simulink subsystem "ApplicationMotorSwapHighPrio"  (R2024b)
settings: Solver=VariableStepAuto  StartTime=0.0  StopTime=10.0  RelTol=1e-3
values from neighbouring files (symbols this model uses):
  Ts = T_pwm    [mcbMotorSwapData.m]
undefined symbols (not defined in the file or in its folder): inverter, NumBits1, NumBits2, Per, pmsm, PosRange1, PosRange2, Slope1, Slope2, Unit
libraries: simulink x17, mcbcontrolslib x4, mcbpmsmparamestlib x3, mcbfoclib x2, mcbpmsmiflib x2, mcbpositiondecoderlib x2, mcbcomputeparameterlib x1, mcbcontrollergainlib x1
(part 1 of 2)
settings Model: Creator=The MathWorks, Inc.  LastModifiedBy=snarayan
settings RTWCC: GPUComputeCapability=3.5

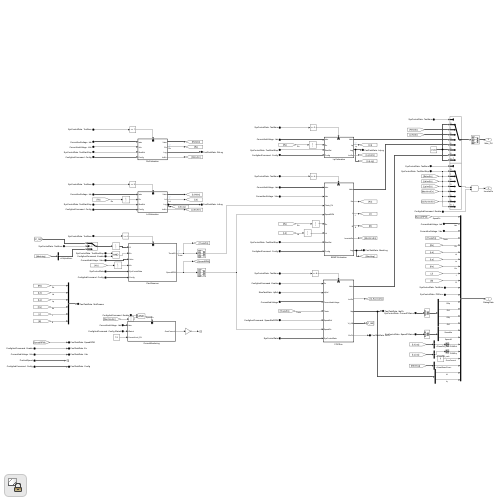
[thumbnail: Simulink's stored preview of the top-level diagram]
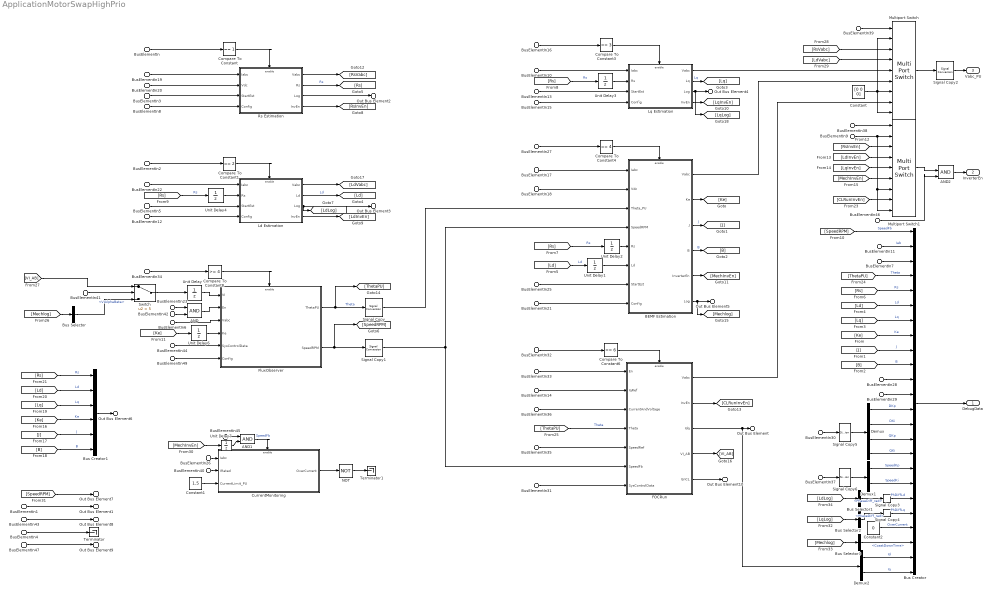
== system ApplicationMotorSwapHighPrio ==
  BusElementIn{1,33,42,45..46} (5 alike) : Inport  PortName=ConfigAndCommand  Element=Enable
  BusElementIn{8,12,15,21,47,49} (6 alike) : Inport  PortName=ConfigAndCommand  Element=Config
  BusElementIn40 : Inport  PortName=ConfigAndCommand  Element=Config.IRated
  BusElementIn35 : Inport  PortName=ConfigAndCommand  Element=SpeedRefRPM
  BusElementIn36 : Inport  Port=2  PortName=CurrentAndVoltage
  BusElementIn{10..11,17,19,22,26} (6 alike) : Inport  Port=2  PortName=CurrentAndVoltage  Element=Iab
  BusElementIn{7,18,20,43} (4 alike) : Inport  Port=2  PortName=CurrentAndVoltage  Element=Vdc
  BusElementIn6 : Inport  Port=2  PortName=CurrentAndVoltage  Element=Vabc
  BusElementIn4 : Inport  Port=3  PortName=PosAndSpeed
  BusElementIn14 : Inport  Port=4  PortName=SlowTaskData  Element=IqRef
  BusElementIn31 : Inport  Port=5  PortName=SysControlData
  BusElementIn44 : Inport  Port=5  PortName=SysControlData
  BusElementIn{,2,16,27..28,32,34,38..39,41} (10 alike) : Inport  Port=5  PortName=SysControlData  Element=TestNum
  BusElementIn29 : Inport  Port=5  PortName=SysControlData  Element=PEError
  BusElementIn{3,5,9,13,23,25} (6 alike) : Inport  Port=5  PortName=SysControlData  Element=TestStartStop
  BusElementIn30 : Inport  Port=5  PortName=SysControlData  Element=CurrentPIGains
  BusElementIn37 : Inport  Port=5  PortName=SysControlData  Element=SpeedPIGains
  AND : Logic  AllPortsSameDT=off  OutDataTypeStr=boolean
  AND1 : Logic  AllPortsSameDT=off  OutDataTypeStr=boolean
  AND2 : Logic  IconShape=distinctive  AllPortsSameDT=off  OutDataTypeStr=boolean
  BEMF Estimation : Subsystem
  Bus Creator : BusCreator  Inputs=24
  Bus Creator1 : BusCreator  Inputs=6
  Bus Selector : BusSelector  OutputSignals=VIAlphaBeta
  Bus Selector1 : BusSelector  OutputSignals=PhaseDiff_rad
  Bus Selector2 : BusSelector  OutputSignals=PhaseDiff_rad
  Bus Selector3 : BusSelector  OutputSignals=CoastDownTime
  Compare To Constant : simulink/Logic and Bit Operations/Compare To Constant  relop===  const=1  OutDataTypeStr=boolean
  Compare To Constant1 : simulink/Logic and Bit Operations/Compare To Constant  relop===  const=2  OutDataTypeStr=boolean
  Compare To Constant3 : simulink/Logic and Bit Operations/Compare To Constant  relop===  const=3  OutDataTypeStr=boolean
  Compare To Constant4 : simulink/Logic and Bit Operations/Compare To Constant  relop===  const=4  OutDataTypeStr=boolean
  Compare To Constant6 : simulink/Logic and Bit Operations/Compare To Constant  relop===  const=6  OutDataTypeStr=boolean
  Compare To Constant8 : simulink/Logic and Bit Operations/Compare To Constant  relop=>=  const=4  OutDataTypeStr=boolean
  Constant : Constant  Value=[0 0 0]  OutDataTypeStr=dataType
  Constant1 : Constant  Value=1.5  OutDataTypeStr=dataType
  Constant2 : Constant  Value=0  OutDataTypeStr=single
  CurrentMonitoring : Subsystem
  Demux : Demux
  Demux1 : Demux  Outputs=2
  Demux2 : Demux  Outputs=2
  FOCRun : Subsystem  TreatAsAtomicUnit=on
  FluxObserver : Subsystem
  Ld Estimation : Subsystem
  Lq Estimation : Subsystem
  Multiport Switch : MultiPortSwitch  DataPortOrder=Zero-based contiguous  Inputs=8  DiagnosticForDefault=None  zeroidx=on  SaturateOnIntegerOverflow=off  InputSameDT=off
  Multiport Switch1 : MultiPortSwitch  DataPortOrder=Zero-based contiguous  Inputs=8  DiagnosticForDefault=None  zeroidx=on  SaturateOnIntegerOverflow=off  InputSameDT=off
  NOT : Logic  Operator=NOT  IconShape=distinctive  AllPortsSameDT=off  OutDataTypeStr=boolean
  Rs Estimation : Subsystem
  Signal Copy{,1..6} (7 alike) : SignalConversion  OverrideOpt=on
  Switch : Switch  Criteria=u2 > Threshold  Threshold=5  SaturateOnIntegerOverflow=off  InputSameDT=off
  Terminator : Terminator
  Terminator1 : Terminator
  Unit Delay{,1..4,6..7} (7 alike) : UnitDelay  SampleTime=-1  HasFrameUpgradeWarning=on
  DebugData : Outport
  InverterEn : Outport  Port=2
  Vabc_PU : Outport  Port=3
  Out Bus Element : Outport  Port=4  PortName=FastTaskData  Element=IdqFb
  Out Bus Element1 : Outport  Port=4  PortName=FastTaskData  Element=En
  Out Bus Element2 : Outport  Port=4  PortName=FastTaskData  Element=RsLog
  Out Bus Element3 : Outport  Port=4  PortName=FastTaskData  Element=LdLog
  Out Bus Element4 : Outport  Port=4  PortName=FastTaskData  Element=LqLog
  Out Bus Element5 : Outport  Port=4  PortName=FastTaskData  Element=MechLog
  Out Bus Element6 : Outport  Port=4  PortName=FastTaskData  Element=MotParams
  Out Bus Element7 : Outport  Port=4  PortName=FastTaskData  Element=SpeedRPM
  Out Bus Element8 : Outport  Port=4  PortName=FastTaskData  Element=Vdc
  Out Bus Element9 : Outport  Port=4  PortName=FastTaskData  Element=Config
  Out Bus Element10 : Outport  Port=4  PortName=FastTaskData  Element=EnCL
  wires:
  Bus Creator/1 -> DebugData/1
  BusElementIn19/1 -> Rs Estimation/1(Iabc)
  BusElementIn20/1 -> Rs Estimation/2(Vdc)
  [Rs] -> Bus Creator/5  "Rs"
  FOCRun/3(Idq) -> Out Bus Element/1, Demux2/1
  BusElementIn11/1 -> Bus Creator/2  "Iab"
  BusElementIn14/1 -> FOCRun/2(IqRef)
  Rs Estimation/3(Log) -> Out Bus Element2/1
  BusElementIn1/1 -> Out Bus Element1/1
  BusElementIn/1 -> Compare To Constant/1
  BusElementIn22/1 -> Ld Estimation/1(Iabc)
  BusElementIn5/1 -> Ld Estimation/3(StartEst)
  BusElementIn12/1 -> Ld Estimation/4(Config)
  Ld Estimation/3(Log) -> [LdLog], Out Bus Element3/1
  Compare To Constant1/1 -> Ld Estimation/Enable
  BusElementIn2/1 -> Compare To Constant1/1
  BusElementIn3/1 -> Rs Estimation/3(StartEst)
  BusElementIn10/1 -> Lq Estimation/1(Iabc)
  BusElementIn13/1 -> Lq Estimation/3(StartEst)
  BusElementIn15/1 -> Lq Estimation/4(Config)
  Lq Estimation/3(Log) -> Out Bus Element4/1, [LqLog]
  Compare To Constant3/1 -> Lq Estimation/Enable
  BusElementIn16/1 -> Compare To Constant3/1
  [Ld] -> Bus Creator/6  "Ld"
  [Lq] -> Bus Creator/7  "Lq"
  FluxObserver/1(ThetaPU) -> Signal Copy/1, [ThetaPU]  "Theta"
  BusElementIn17/1 -> BEMF Estimation/1(Iabc)
  BusElementIn18/1 -> BEMF Estimation/2(Vdc)
  Unit Delay1/1 -> BEMF Estimation/6(Ld)
  BusElementIn25/1 -> BEMF Estimation/7(StartEst)
  BusElementIn21/1 -> BEMF Estimation/8(Config)
  [Ke] -> Bus Creator/8  "Ke"
  [J] -> Bus Creator/9  "J"
  [B] -> Bus Creator/10  "B"
  BEMF Estimation/6(Log) -> Out Bus Element5/1, [Mechlog]
  Compare To Constant4/1 -> BEMF Estimation/Enable
  BusElementIn27/1 -> Compare To Constant4/1
  BEMF Estimation/2(Ke) -> [Ke]
  BEMF Estimation/3(J) -> [J]  "J"
  BEMF Estimation/4(B) -> [B]  "B"
  Lq Estimation/2(Lq) -> [Lq]  "Lq"
  Ld Estimation/2(Ld) -> [Ld]  "Ld"
  [Ld] -> Unit Delay1/1  "Ld"
  Rs Estimation/2(Rs) -> [Rs]  "Rs"
  Unit Delay2/1 -> BEMF Estimation/5(Rs)
  [Rs] -> Unit Delay2/1  "Rs"
  Unit Delay3/1 -> Lq Estimation/2(Rs)
  [Rs] -> Unit Delay3/1  "Rs"
  Unit Delay4/1 -> Ld Estimation/2(Rs)
  [Rs] -> Unit Delay4/1  "Rs"
  FluxObserver/2(SpeedRPM) -> Signal Copy1/1, [SpeedRPM]
  BusElementIn9/1 -> Multiport Switch1/2, Multiport Switch1/7, Multiport Switch1/9
  Rs Estimation/4(InvEn) -> [RsInvEn]
  Ld Estimation/4(InvEn) -> [LdInvEn]
  Lq Estimation/4(InvEn) -> [LqInvEn]
  BEMF Estimation/5(InverterEn) -> [MechInvEn]
  BusElementIn28/1 -> Bus Creator/11
  BusElementIn29/1 -> Bus Creator/12
  [Ld] -> Bus Creator1/2  "Ld"
  [Lq] -> Bus Creator1/3  "Lq"
  [Rs] -> Bus Creator1/1  "Rs"
  [Ke] -> Bus Creator1/4  "Ke"
  [J] -> Bus Creator1/5  "J"
  [B] -> Bus Creator1/6  "B"
  Bus Creator1/1 -> Out Bus Element6/1
  Compare To Constant6/1 -> FOCRun/Enable
  BusElementIn32/1 -> Compare To Constant6/1
  FOCRun/2(InvEn) -> [CLRunInvEn]
  BusElementIn33/1 -> FOCRun/1(En)
  [ThetaPU] -> FOCRun/4(Theta)  "Theta"
  BusElementIn4/1 -> Terminator/1
  Unit Delay/1 -> FluxObserver/1(VI)
  BusElementIn23/1 -> AND/1
  [Mechlog] -> Bus Selector/1
  BusElementIn34/1 -> Compare To Constant8/1
  Compare To Constant8/1 -> FluxObserver/Enable
  Signal Copy/1 -> BEMF Estimation/3(Theta_PU)
  Signal Copy1/1 -> FOCRun/6(SpeedFb), BEMF Estimation/4(SpeedRPM)
  AND/1 -> FluxObserver/2(En)
  Switch/1 -> Unit Delay/1
  FOCRun/4(VI_AB) -> [VI_AB]
  [VI_AB] -> Switch/1
  Bus Selector/1 -> Switch/3  "<VIAlphaBeta>"
  BusElementIn41/1 -> Switch/2
  BusElementIn42/1 -> AND/2
  BusElementIn43/1 -> Out Bus Element8/1
  BusElementIn31/1 -> FOCRun/7(SysControlData)
  BusElementIn36/1 -> FOCRun/3(CurrentAndVoltage)
  [SpeedRPM] -> Out Bus Element7/1
  BusElementIn35/1 -> FOCRun/5(SpeedRef)
  BusElementIn7/1 -> Bus Creator/3
  Ld Estimation/1(Vabc) -> [LdVabc]
  FOCRun/1(Vabc) -> Multiport Switch/8
  BusElementIn30/1 -> Signal Copy5/1
  Demux/3 -> Bus Creator/15  "QKp"
  Demux/4 -> Bus Creator/16  "QKi"
  Demux/2 -> Bus Creator/14  "DKi"
  Demux/1 -> Bus Creator/13  "DKp"
  Demux1/1 -> Bus Creator/17  "SpeedKp"
  Demux1/2 -> Bus Creator/18  "SpeedKi"
  BusElementIn37/1 -> Signal Copy6/1
  Compare To Constant/1 -> Rs Estimation/Enable
  BusElementIn39/1 -> Multiport Switch/1
  Constant/1 -> Multiport Switch/7, Multiport Switch/9, Multiport Switch/2
  Multiport Switch/1 -> Signal Copy2/1
  Rs Estimation/1(Vabc) -> [RsVabc]
  [LdVabc] -> Multiport Switch/4
  [RsVabc] -> Multiport Switch/3
  Lq Estimation/1(Vabc) -> Multiport Switch/5
  BEMF Estimation/1(Vabc) -> Multiport Switch/6
  BusElementIn38/1 -> Multiport Switch1/1
  [RsInvEn] -> Multiport Switch1/3
  [LdInvEn] -> Multiport Switch1/4
  [LqInvEn] -> Multiport Switch1/5
  [MechInvEn] -> Multiport Switch1/6
  [CLRunInvEn] -> Multiport Switch1/8
  BusElementIn6/1 -> FluxObserver/3(Vabc)
  Unit Delay6/1 -> FluxObserver/4(Ke)
  [Ke] -> Unit Delay6/1
  BusElementIn44/1 -> FluxObserver/5(SysControlData)
  BusElementIn8/1 -> Rs Estimation/4(Config)
  BusElementIn26/1 -> CurrentMonitoring/1(Iabc)
  BusElementIn40/1 -> CurrentMonitoring/2(IRated)
  Constant1/1 -> CurrentMonitoring/3(CurrentLimit_PU)
  CurrentMonitoring/1(OverCurrent) -> NOT/1
  Unit Delay7/1 -> AND1/2
  BusElementIn45/1 -> AND1/1
  [MechInvEn] -> Unit Delay7/1
  AND2/1 -> InverterEn/1
  Multiport Switch1/1 -> AND2/1
  BusElementIn46/1 -> AND2/2
  BusElementIn47/1 -> Out Bus Element9/1
  Signal Copy2/1 -> Vabc_PU/1
  BusElementIn49/1 -> FluxObserver/6(Config)
  [LdLog] -> Bus Selector1/1
  Bus Selector1/1 -> Signal Copy3/1  "<PhaseDiff_rad>"
  [LqLog] -> Bus Selector2/1
  Signal Copy3/1 -> Bus Creator/19  "PhDiffLd"
  Bus Selector2/1 -> Signal Copy4/1  "<PhaseDiff_rad>"
  Signal Copy4/1 -> Bus Creator/20  "PhDiffLq"
  AND1/1 -> CurrentMonitoring/Enable  "SpeedFb"
  [SpeedRPM] -> Bus Creator/1  "SpeedFb"
  NOT/1 -> Terminator1/1
  Constant2/1 -> Bus Creator/21  "OverCurrent"
  [Mechlog] -> Bus Selector3/1
  Bus Selector3/1 -> Bus Creator/22  "<CoastDownTime>"
  Demux2/2 -> Bus Creator/24  "Iq"
  Demux2/1 -> Bus Creator/23  "Id"
  FOCRun/5(EnCL) -> Out Bus Element10/1
  [ThetaPU] -> Bus Creator/4  "Theta"
  Signal Copy5/1 -> Demux/1
  Signal Copy6/1 -> Demux1/1

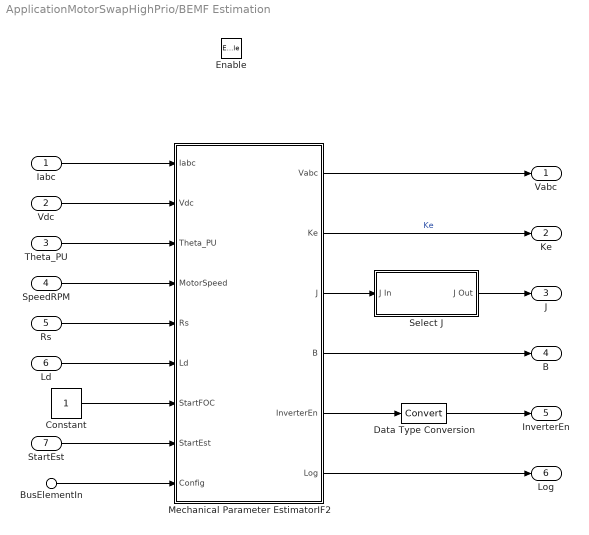
== system ApplicationMotorSwapHighPrio/BEMF Estimation ==
  Iabc : Inport
  Vdc : Inport  Port=2
  Theta_PU : Inport  Port=3
  SpeedRPM : Inport  Port=4
  Rs : Inport  Port=5
  Ld : Inport  Port=6
  StartEst : Inport  Port=7
  BusElementIn : Inport  Port=8  PortName=Config
  Enable : EnablePort  StatesWhenEnabling=reset
  Constant : Constant  OutDataTypeStr=Inherit: Inherit via back propagation
  Data Type Conversion : DataTypeConversion  SaturateOnIntegerOverflow=off  RndMeth=Floor
  Mechanical Parameter EstimatorIF2 : Subsystem  AncestorBlock=mcblib/Parameter Estimation/PMSM Parameter Estimation/Mechanical Parameter Estimator  InitFcn=|  mask(PMSM Mechanical Parameter Estimator){}
      | mcb.internal.manageMCBResource('register',gcbh);
      | mcb.internal.logDDUXData;
      mask help: mcb:ParamEstLib:PmsmKeJBEstBlkDlgDes
      mask init:
      | % mcb.internal.PMSMParameterEstimationCb();
      settings: LibrarySourceBlock=mcblib/Parameter Estimation/PMSM Parameter Estimation/Mechanical Parameter Estimator
      mask Help: eval('mcb_helpview(''pmsmmechanicalparameterestimator'')')
      mask DialogControl DescGroupVar Prompt: mcb:ParamEstLib:PmsmKeJBEstBlkDlgTitle
      mask Display:
      | fprintf('PMSM\nMechanical\nParameter\nEstimator');
      | port_label('input',1,'Iabc');
      | port_label('input',2,'Vdc');
      | port_label('input',3,'Theta');
      | port_label('input',4,'Speed');
      | port_label('input',5,'Rs');
      | port_label('input',6,'Ld');
      | port_label('input',7,'StartFOC');
      | port_label('input',8,'StartStop');
      | port_label('input',9,'Config');
      | 
      | port_label('output',1,'Vabc');
      | port_label('output',2,'Ke');
      | port_label('output',3,'J');
      | port_label('output',4,'B');
      | port_label('output',5,'InverterEn');
      | port_label('output',6,'Log');
  Select J : Subsystem  Variant=on  VariantControlMode=sim codegen switching
  Vabc : Outport
  Ke : Outport  Port=2  InitialOutput=pmsm.Ke
  J : Outport  Port=3  InitialOutput=pmsm.J
  B : Outport  Port=4  InitialOutput=pmsm.B
  InverterEn : Outport  Port=5  InitialOutput=true
  Log : Outport  Port=6
  wires:
  Constant/1 -> Mechanical Parameter EstimatorIF2/7(StartFOC)
  Mechanical Parameter EstimatorIF2/3(J) -> Select J/1(J In)
  Mechanical Parameter EstimatorIF2/4(B) -> B/1
  Select J/1(J Out) -> J/1
  Data Type Conversion/1 -> InverterEn/1
  Mechanical Parameter EstimatorIF2/6(Log) -> Log/1
  Mechanical Parameter EstimatorIF2/2(Ke) -> Ke/1  "Ke"
  Mechanical Parameter EstimatorIF2/5(InverterEn) -> Data Type Conversion/1
  Mechanical Parameter EstimatorIF2/1(Vabc) -> Vabc/1
  BusElementIn/1 -> Mechanical Parameter EstimatorIF2/9(Config)
  StartEst/1 -> Mechanical Parameter EstimatorIF2/8(StartEst)
  Ld/1 -> Mechanical Parameter EstimatorIF2/6(Ld)
  Rs/1 -> Mechanical Parameter EstimatorIF2/5(Rs)
  SpeedRPM/1 -> Mechanical Parameter EstimatorIF2/4(MotorSpeed)
  Theta_PU/1 -> Mechanical Parameter EstimatorIF2/3(Theta_PU)
  Vdc/1 -> Mechanical Parameter EstimatorIF2/2(Vdc)
  Iabc/1 -> Mechanical Parameter EstimatorIF2/1(Iabc)

== system ApplicationMotorSwapHighPrio/CurrentMonitoring ==
  Iabc : Inport
  IRated : Inport  Port=2
  CurrentLimit_PU : Inport  Port=3
  Enable : EnablePort  StatesWhenEnabling=reset
  Current and Voltage Monitoring : Subsystem
  NOT : Logic  Operator=NOT  IconShape=distinctive  AllPortsSameDT=off  OutDataTypeStr=boolean
  Unit Delay : UnitDelay  SampleTime=-1  HasFrameUpgradeWarning=on
  OverCurrent : Outport  InitialOutput=0
  wires:
  IRated/1 -> Current and Voltage Monitoring/2(IRated)
  Iabc/1 -> Current and Voltage Monitoring/1(Iabc)
  Current and Voltage Monitoring/1(OverCurrent) -> NOT/1, OverCurrent/1  "in_oc"
  CurrentLimit_PU/1 -> Current and Voltage Monitoring/3(CurrentLimit)
  NOT/1 -> Unit Delay/1
  Unit Delay/1 -> Current and Voltage Monitoring/Enable

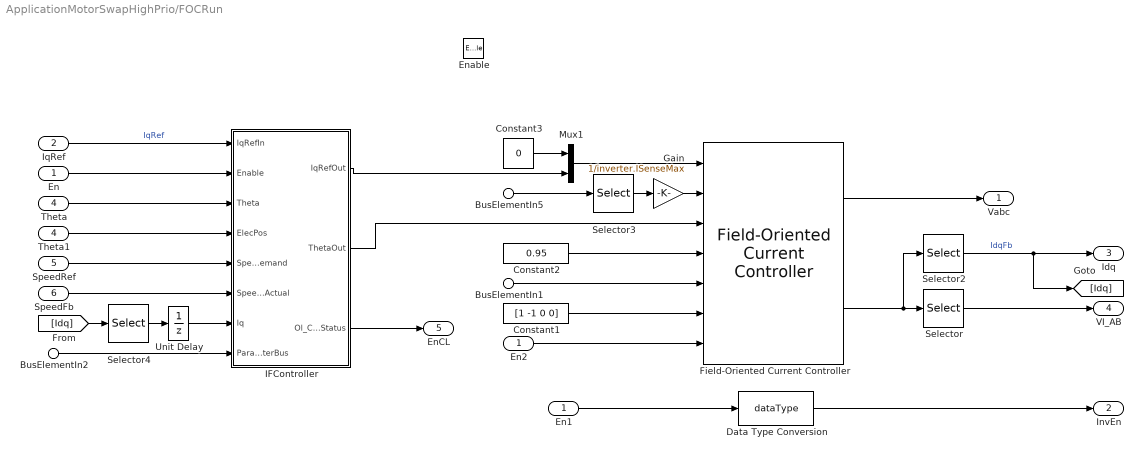
== system ApplicationMotorSwapHighPrio/FOCRun ==
  En : Inport
  IqRef : Inport  Port=2
  BusElementIn5 : Inport  Port=3  PortName=CurrentAndVoltage  Element=Iab
  Theta : Inport  Port=4
  SpeedRef : Inport  Port=5
  SpeedFb : Inport  Port=6
  BusElementIn1 : Inport  Port=7  PortName=SysControlData  Element=CurrentPIGains
  BusElementIn2 : Inport  Port=7  PortName=SysControlData  Element=IFParams
  Enable : EnablePort  StatesWhenEnabling=reset
  Constant1 : Constant  Value=[1 -1 0 0]  OutDataTypeStr=dataType
  Constant2 : Constant  Value=0.95  OutDataTypeStr=dataType
  Constant3 : Constant  Value=0  OutDataTypeStr=single
  Data Type Conversion : DataTypeConversion  OutDataTypeStr=dataType  RndMeth=Simplest  SaturateOnIntegerOverflow=off
  En1 : InportShadow
  En2 : InportShadow
  Field-Oriented Current Controller : mcbfoclib/Field-Oriented Current Controller  AngleUnit=Per-unit  NumberOfLUTPoints=1024  AxisAlignment=D-axis  SaturationMethod=D-Q equivalence  PWMMethod=SVM: space vector modulation
  Gain : Gain  Gain=1/inverter.ISenseMax  RndMeth=Simplest  OutDataTypeStr=Inherit: Same as input
  IFController : Subsystem
  Mux1 : Mux  Inputs=2
  Selector : Selector  InputPortWidth=8  IndexOptions=Index vector (dialog)  Indices=[5 6 7 8]  OutputSizes=1
  Selector2 : Selector  InputPortWidth=8  IndexOptions=Index vector (dialog)  Indices=[1 2]  OutputSizes=1
  Selector3 : Selector  InputPortWidth=3  IndexOptions=Index vector (dialog)  Indices=[1 2]  OutputSizes=1
  Selector4 : Selector  InputPortWidth=2  IndexOptions=Index vector (dialog)  Indices=[2]  OutputSizes=1
  Theta1 : InportShadow  Port=4
  Unit Delay : UnitDelay  SampleTime=-1  HasFrameUpgradeWarning=on
  Vabc : Outport
  InvEn : Outport  Port=2
  Idq : Outport  Port=3
  VI_AB : Outport  Port=4
  EnCL : Outport  Port=5
  wires:
  IFController/3(Ol_CL_Status) -> EnCL/1
  IFController/2(ThetaOut) -> Field-Oriented Current Controller/3
  IFController/1(IqRefOut) -> Mux1/2
  BusElementIn2/1 -> IFController/8(ParamterBus)
  Unit Delay/1 -> IFController/7(Iq)
  SpeedFb/1 -> IFController/6(SpeedActual)
  SpeedRef/1 -> IFController/5(SpeedDemand)
  Theta1/1 -> IFController/4(ElecPos)
  Theta/1 -> IFController/3(Theta)
  En/1 -> IFController/2(Enable)
  IqRef/1 -> IFController/1(IqRefIn)  "IqRef"
  BusElementIn1/1 -> Field-Oriented Current Controller/5
  Constant3/1 -> Mux1/1
  Mux1/1 -> Field-Oriented Current Controller/1
  Field-Oriented Current Controller/1 -> Vabc/1
  En2/1 -> Field-Oriented Current Controller/7
  Constant1/1 -> Field-Oriented Current Controller/6
  Selector4/1 -> Unit Delay/1
  [Idq] -> Selector4/1
  Selector/1 -> VI_AB/1
  BusElementIn5/1 -> Selector3/1
  Constant2/1 -> Field-Oriented Current Controller/4
  Selector2/1 -> [Idq], Idq/1  "IdqFb"
  Field-Oriented Current Controller/2 -> Selector/1, Selector2/1
  Gain/1 -> Field-Oriented Current Controller/2
  Data Type Conversion/1 -> InvEn/1
  Selector3/1 -> Gain/1
  En1/1 -> Data Type Conversion/1

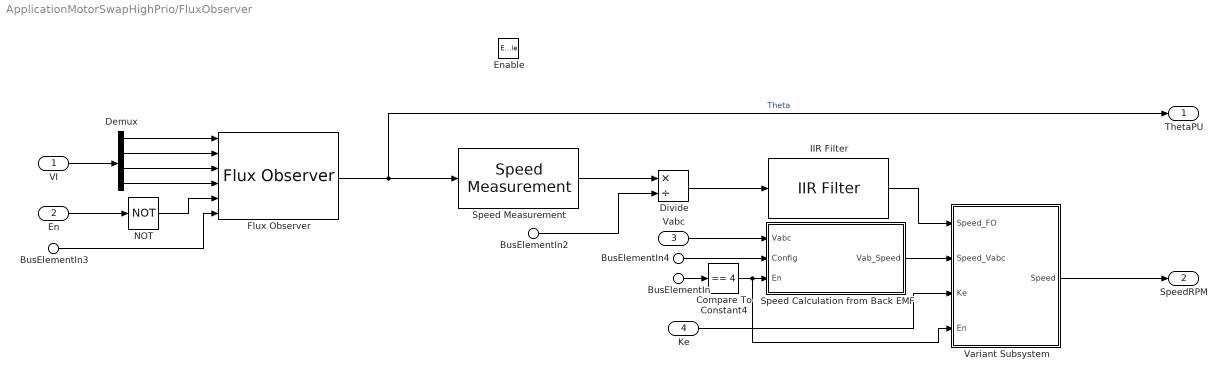
== system ApplicationMotorSwapHighPrio/FluxObserver ==
  VI : Inport
  En : Inport  Port=2
  Vabc : Inport  Port=3
  Ke : Inport  Port=4
  BusElementIn : Inport  Port=5  PortName=SysControlData  Element=TestNum
  BusElementIn3 : Inport  Port=5  PortName=SysControlData  Element=FOParams
  BusElementIn4 : Inport  Port=6  PortName=Config
  BusElementIn2 : Inport  Port=6  PortName=Config  Element=P
  Enable : EnablePort
  Compare To Constant4 : simulink/Logic and Bit Operations/Compare To Constant  relop===  const=4  OutDataTypeStr=boolean
  Demux : Demux
  Divide : Product  Inputs=*/
  Flux Observer : mcbpositiondecoderlib/Flux Observer  MotorSelection=PMSM  DataTypeSelect=off  BlockInputUnit=Per-unit  PerUnitVoltage=inverter.V_dc/sqrt(3)  PerUnitCurrent=inverter.ISenseMax  PositionSelect=on  FluxSelect=off  TorqueSelect=off  PolePairs=4  StatorResistance=0.36  StatorDAxisInductance=0.2e-3  StatorLeakageInductance=0.0068  RotorLeakageInductance=0.0068  MagnetizingInductance=0.0300  CutoffFreq=3.1863  BlockSampleTime=Ts  ParameterBusInput=on  PositionUnit=Per-unit  PositionDatatype=dataType  FluxUnit=Weber  PerUnitFlux=0.1  FluxDatatype=single  TorqueUnit=Nm  PerUnitTorque=100  TorqueDatatype=single  DataType=0
  IIR Filter : mcbcontrolslib/IIR Filter  VariantControl=Low Pass Filter  VariantSelect=Low-pass  FilterConstantInputType=Specify via dialog  Filter_constant=0.01  advancedSettings=on  Ts=Ts  cutOff_freq=25.722
  NOT : Logic  Operator=NOT  IconShape=distinctive  AllPortsSameDT=off  OutDataTypeStr=boolean
  Speed Calculation from Back EMF : Subsystem
  Speed Measurement : mcbpositiondecoderlib/Speed Measurement  PositionUnit=Per unit  PositionScalingDatatype=uint32  SpeedCalculationMode=Time interval for speed calculation  SampleTimeAsync=Ts  MaximumApplicationSpeed=1000  SpeedResolution=5e-6  DelayLength=10  MaximumMeasurableSpeed=47999  MeasurableSpeedResolution=2.2352e-05  SpeedUnit=RPM  PerUnitSpeed=1000  SpeedDataType=dataType
  Variant Subsystem : Subsystem  Variant=on  VariantControlMode=sim codegen switching
  ThetaPU : Outport
  SpeedRPM : Outport  Port=2
  wires:
  Ke/1 -> Variant Subsystem/3(Ke)
  Compare To Constant4/1 -> Speed Calculation from Back EMF/3(En), Variant Subsystem/4(En)
  BusElementIn/1 -> Compare To Constant4/1
  BusElementIn4/1 -> Speed Calculation from Back EMF/2(Config)
  Vabc/1 -> Speed Calculation from Back EMF/1(Vabc)
  Speed Calculation from Back EMF/1(Vab_Speed) -> Variant Subsystem/2(Speed_Vabc)
  IIR Filter/1 -> Variant Subsystem/1(Speed_FO)
  Variant Subsystem/1(Speed) -> SpeedRPM/1
  VI/1 -> Demux/1
  BusElementIn3/1 -> Flux Observer/6
  En/1 -> NOT/1
  NOT/1 -> Flux Observer/5
  Demux/1 -> Flux Observer/1
  Demux/4 -> Flux Observer/4
  Demux/2 -> Flux Observer/2
  Demux/3 -> Flux Observer/3
  BusElementIn2/1 -> Divide/2
  Divide/1 -> IIR Filter/1
  Speed Measurement/1 -> Divide/1
  Flux Observer/1 -> Speed Measurement/1, ThetaPU/1  "Theta"

== system ApplicationMotorSwapHighPrio/Ld Estimation ==
  Iabc : Inport
  Rs : Inport  Port=2
  StartEst : Inport  Port=3
  Config : Inport  Port=4
  Enable : EnablePort  StatesWhenEnabling=reset
  Ld Estimator : mcbpmsmparamestlib/Ld Estimator
  Vabc : Outport
  Ld : Outport  Port=2  InitialOutput=pmsm.Ld
  Log : Outport  Port=3
  InvEn : Outport  Port=4
  wires:
  Ld Estimator/2 -> Ld/1  "Ld"
  Config/1 -> Ld Estimator/4
  Ld Estimator/1 -> Vabc/1
  Rs/1 -> Ld Estimator/2
  Ld Estimator/3 -> Log/1
  StartEst/1 -> Ld Estimator/3, InvEn/1
  Iabc/1 -> Ld Estimator/1

== system ApplicationMotorSwapHighPrio/Lq Estimation ==
  Iabc : Inport
  Rs : Inport  Port=2
  StartEst : Inport  Port=3
  Config : Inport  Port=4
  Enable : EnablePort  StatesWhenEnabling=reset
  Lq Estimator : mcbpmsmparamestlib/Lq Estimator
  Vabc : Outport
  Lq : Outport  Port=2  InitialOutput=pmsm.Lq
  Log : Outport  Port=3
  InvEn : Outport  Port=4
  wires:
  StartEst/1 -> Lq Estimator/3, InvEn/1
  Lq Estimator/3 -> Log/1
  Rs/1 -> Lq Estimator/2
  Lq Estimator/1 -> Vabc/1
  Config/1 -> Lq Estimator/4
  Lq Estimator/2 -> Lq/1
  Iabc/1 -> Lq Estimator/1

== system ApplicationMotorSwapHighPrio/Rs Estimation ==
  Iabc : Inport
  Vdc : Inport  Port=2
  StartEst : Inport  Port=3
  Config : Inport  Port=4
  Enable : EnablePort  StatesWhenEnabling=reset
  Rs Estimator : mcbpmsmparamestlib/Rs Estimator
  Vabc : Outport
  Rs : Outport  Port=2  InitialOutput=pmsm.Rs
  Log : Outport  Port=3
  InvEn : Outport  Port=4
  wires:
  Rs Estimator/1 -> Vabc/1
  Iabc/1 -> Rs Estimator/1
  Rs Estimator/3 -> Log/1
  Vdc/1 -> Rs Estimator/2
  Config/1 -> Rs Estimator/4
  StartEst/1 -> InvEn/1, Rs Estimator/3
  Rs Estimator/2 -> Rs/1  "Rs"

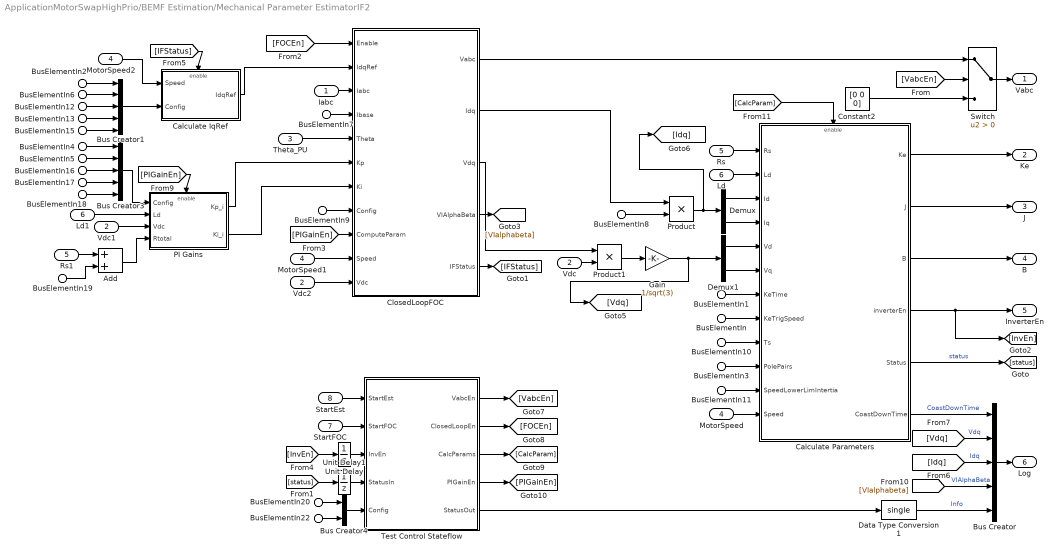
== system ApplicationMotorSwapHighPrio/BEMF Estimation/Mechanical Parameter EstimatorIF2 ==
  Iabc : Inport  OutDataTypeStr=single
  Vdc : Inport  Port=2  OutDataTypeStr=single
  Theta_PU : Inport  Port=3  OutDataTypeStr=single
  MotorSpeed : Inport  Port=4  OutDataTypeStr=single
  Rs : Inport  Port=5  OutDataTypeStr=single
  Ld : Inport  Port=6  OutDataTypeStr=single
  StartFOC : Inport  Port=7
  StartEst : Inport  Port=8
  BusElementIn9 : Inport  Port=9  PortName=Config
  BusElementIn10 : Inport  Port=9  PortName=Config  Element=Ts
  BusElementIn16 : Inport  Port=9  PortName=Config  Element=Ts
  BusElementIn20 : Inport  Port=9  PortName=Config  Element=Ts
  BusElementIn4 : Inport  Port=9  PortName=Config  Element=Kp
  BusElementIn5 : Inport  Port=9  PortName=Config  Element=Ki
  BusElementIn6 : Inport  Port=9  PortName=Config  Element=IRated
  BusElementIn1 : Inport  Port=9  PortName=Config  Element=KeTime
  BusElementIn22 : Inport  Port=9  PortName=Config  Element=KeTime
  BusElementIn3 : Inport  Port=9  PortName=Config  Element=P
  BusElementIn11 : Inport  Port=9  PortName=Config  Element=JSpeedLow
  BusElementIn2 : Inport  Port=9  PortName=Config  Element=IqRefFoc
  BusElementIn{7..8,12,18} (4 alike) : Inport  Port=9  PortName=Config  Element=ImaxInverter
  BusElementIn : Inport  Port=9  PortName=Config  Element=KeSpeed
  BusElementIn13 : Inport  Port=9  PortName=Config  Element=KeSpeed
  BusElementIn15 : Inport  Port=9  PortName=Config  Element=NRated
  BusElementIn17 : Inport  Port=9  PortName=Config  Element=KpKiInputEnable
  BusElementIn19 : Inport  Port=9  PortName=Config  Element=RBoard
  Add : Sum  RndMeth=Simplest  OutDataTypeStr=Inherit: Same as first input
  Bus Creator : BusCreator  Inputs=5
  Bus Creator1 : BusCreator  Inputs=5
  Bus Creator3 : BusCreator  Inputs=5
  Bus Creator4 : BusCreator  Inputs=2
  Calculate IqRef : Subsystem
  Calculate Parameters : Subsystem
  ClosedLoopFOC : Subsystem
  Constant2 : Constant  Value=[0 0 0]  OutDataTypeStr=single
  Data Type Conversion1 : DataTypeConversion  OutDataTypeStr=single  RndMeth=Simplest  SaturateOnIntegerOverflow=off
  Demux : Demux  Outputs=2
  Demux1 : Demux  Outputs=2
  Gain : Gain  Gain=1/sqrt(3)  RndMeth=Simplest  OutDataTypeStr=Inherit: Same as input
  Ld1 : InportShadow  Port=6  OutDataTypeStr=single
  MotorSpeed1 : InportShadow  Port=4  OutDataTypeStr=single
  MotorSpeed2 : InportShadow  Port=4  OutDataTypeStr=single
  PI Gains : Subsystem
  Product : Product  RndMeth=Simplest  OutDataTypeStr=Inherit: Same as first input
  Product1 : Product  RndMeth=Simplest  OutDataTypeStr=Inherit: Same as first input
  Rs1 : InportShadow  Port=5  OutDataTypeStr=single
  Switch : Switch  Criteria=u2 > Threshold  SaturateOnIntegerOverflow=off  InputSameDT=off
  Test Control Stateflow : Subsystem
  Unit Delay : UnitDelay  SampleTime=-1  HasFrameUpgradeWarning=on
  Unit Delay1 : UnitDelay  SampleTime=-1  HasFrameUpgradeWarning=on
  Vdc1 : InportShadow  Port=2  OutDataTypeStr=single
  Vdc2 : InportShadow  Port=2  OutDataTypeStr=single
  Vabc : Outport  InitialOutput=[0 0 0]
  Ke : Outport  Port=2
  J : Outport  Port=3
  B : Outport  Port=4
  InverterEn : Outport  Port=5
  Log : Outport  Port=6
  wires:
  Data Type Conversion1/1 -> Bus Creator/5  "Info"
  [PIGainEn] -> PI Gains/Enable
  Test Control Stateflow/4(PIGainEn) -> [PIGainEn]
  Test Control Stateflow/2(ClosedLoopEn) -> [FOCEn]
  Iabc/1 -> ClosedLoopFOC/3(Iabc)
  [Vdq] -> Bus Creator/2  "Vdq"
  [Idq] -> Bus Creator/3  "Idq"
  BusElementIn19/1 -> Add/2
  Rs1/1 -> Add/1
  Add/1 -> PI Gains/4(Rtotal)
  Vdc1/1 -> PI Gains/3(Vdc)
  Ld1/1 -> PI Gains/2(Ld)
  BusElementIn18/1 -> Bus Creator3/5
  [VabcEn] -> Switch/2
  [InvEn] -> Unit Delay/1
  BusElementIn/1 -> Calculate Parameters/8(KeTrigSpeed)
  ClosedLoopFOC/4(VIAlphaBeta) -> [VIalphabeta]
  Calculate Parameters/6(CoastDownTime) -> Bus Creator/1  "CoastDownTime"
  BusElementIn11/1 -> Calculate Parameters/11(SpeedLowerLimIntertia)
  Calculate Parameters/4(inverterEn) -> InverterEn/1, [InvEn]
  Rs/1 -> Calculate Parameters/1(Rs)
  Calculate Parameters/3(B) -> B/1
  BusElementIn10/1 -> Calculate Parameters/9(Ts)
  Bus Creator/1 -> Log/1
  Calculate Parameters/5(Status) -> [status]  "status"
  Demux/2 -> Calculate Parameters/4(Iq)
  BusElementIn1/1 -> Calculate Parameters/7(KeTime)
  Calculate Parameters/2(J) -> J/1
  Ld/1 -> Calculate Parameters/2(Ld)
  Demux1/2 -> Calculate Parameters/6(Vq)
  Demux1/1 -> Calculate Parameters/5(Vd)
  Demux/1 -> Calculate Parameters/3(Id)
  MotorSpeed/1 -> Calculate Parameters/12(Speed)
  BusElementIn3/1 -> Calculate Parameters/10(PolePairs)
  Calculate Parameters/1(Ke) -> Ke/1
  ClosedLoopFOC/2(Idq) -> Product/1
  Product/1 -> Demux/1, [Idq]
  Vdc/1 -> Product1/2
  ClosedLoopFOC/3(Vdq) -> Product1/1
  Product1/1 -> Gain/1
  Gain/1 -> Demux1/1, [Vdq]
  Theta_PU/1 -> ClosedLoopFOC/5(Theta)
  Switch/1 -> Vabc/1
  Constant2/1 -> Switch/3
  MotorSpeed2/1 -> Calculate IqRef/1(Speed)
  Calculate IqRef/1(IdqRef) -> ClosedLoopFOC/2(IdqRef)
  PI Gains/1(Kp_i) -> ClosedLoopFOC/6(Kp)
  PI Gains/2(Ki_i) -> ClosedLoopFOC/7(Ki)
  BusElementIn12/1 -> Bus Creator1/3
  BusElementIn13/1 -> Bus Creator1/4
  BusElementIn6/1 -> Bus Creator1/2
  BusElementIn2/1 -> Bus Creator1/1
  BusElementIn15/1 -> Bus Creator1/5
  Bus Creator1/1 -> Calculate IqRef/2(Config)
  BusElementIn8/1 -> Product/2
  BusElementIn4/1 -> Bus Creator3/1
  BusElementIn5/1 -> Bus Creator3/2
  BusElementIn16/1 -> Bus Creator3/3
  BusElementIn17/1 -> Bus Creator3/4
  Bus Creator3/1 -> PI Gains/1(Config)
  BusElementIn7/1 -> ClosedLoopFOC/4(Ibase)
  StartEst/1 -> Test Control Stateflow/1(StartEst)
  StartFOC/1 -> Test Control Stateflow/2(StartFOC)
  Unit Delay/1 -> Test Control Stateflow/3(InvEn)
  [status] -> Unit Delay1/1
  Unit Delay1/1 -> Test Control Stateflow/4(StatusIn)
  Bus Creator4/1 -> Test Control Stateflow/5(Config)
  BusElementIn22/1 -> Bus Creator4/2
  BusElementIn20/1 -> Bus Creator4/1
  Test Control Stateflow/5(StatusOut) -> Data Type Conversion1/1
  Test Control Stateflow/1(VabcEn) -> [VabcEn]
  [FOCEn] -> ClosedLoopFOC/1(Enable)
  Test Control Stateflow/3(CalcParams) -> [CalcParam]
  [CalcParam] -> Calculate Parameters/Enable
  BusElementIn9/1 -> ClosedLoopFOC/8(Config)
  [VIalphabeta] -> Bus Creator/4  "VIAlphaBeta"
  ClosedLoopFOC/1(Vabc) -> Switch/1
  [PIGainEn] -> ClosedLoopFOC/9(ComputeParam)
  MotorSpeed1/1 -> ClosedLoopFOC/10(Speed)
  Vdc2/1 -> ClosedLoopFOC/11(Vdc)
  ClosedLoopFOC/5(IFStatus) -> [IFStatus]
  [IFStatus] -> Calculate IqRef/Enable

== system ApplicationMotorSwapHighPrio/BEMF Estimation/Select J ==
  note: 1) Add Subsystem or Model blocks as valid variant choices.
      | 2) You cannot connect blocks at this level. At simulation, connectivity is automatically
      | determined, based on the active variant and port name matching.
  J In : Inport
  Codegen : Subsystem  VariantControl=(codegen)
  Sim : Subsystem  VariantControl=(sim)
  J Out : Outport

== system ApplicationMotorSwapHighPrio/CurrentMonitoring/Current and Voltage Monitoring ==
  note: As a ratio of motor rated current
  Iabc : Inport
  IRated : Inport  Port=2
  CurrentLimit : Inport  Port=3
  Enable : EnablePort
  Abs : Abs  SaturateOnIntegerOverflow=off
  Demux : Demux  Outputs=2
  Divide : Product  Inputs=*/  RndMeth=Simplest  OutDataTypeStr=Inherit: Same as first input
  GreaterThan : RelationalOperator  Operator=>  OutDataTypeStr=boolean  RndMeth=Simplest  InputSameDT=off
  GreaterThan1 : RelationalOperator  Operator=>  OutDataTypeStr=boolean  RndMeth=Simplest  InputSameDT=off
  IIR Filter : mcbcontrolslib/IIR Filter  VariantControl=Low Pass Filter  VariantSelect=Low-pass  FilterConstantInputType=Specify via dialog  Filter_constant=0.01  advancedSettings=off  Ts=50e-6  cutOff_freq=32.1525
  OR : Logic  Operator=OR  IconShape=distinctive  AllPortsSameDT=off  OutDataTypeStr=boolean
  Selector : Selector  InputPortWidth=3  IndexOptions=Index vector (dialog)  Indices=[1 2]  OutputSizes=1
  OverCurrent : Outport
  wires:
  Selector/1 -> Divide/1
  Iabc/1 -> Selector/1
  IRated/1 -> Divide/2
  Demux/1 -> GreaterThan/1
  IIR Filter/1 -> Abs/1
  Divide/1 -> IIR Filter/1
  Abs/1 -> Demux/1
  OR/1 -> OverCurrent/1
  Demux/2 -> GreaterThan1/1
  CurrentLimit/1 -> GreaterThan/2, GreaterThan1/2
  GreaterThan/1 -> OR/1
  GreaterThan1/1 -> OR/2

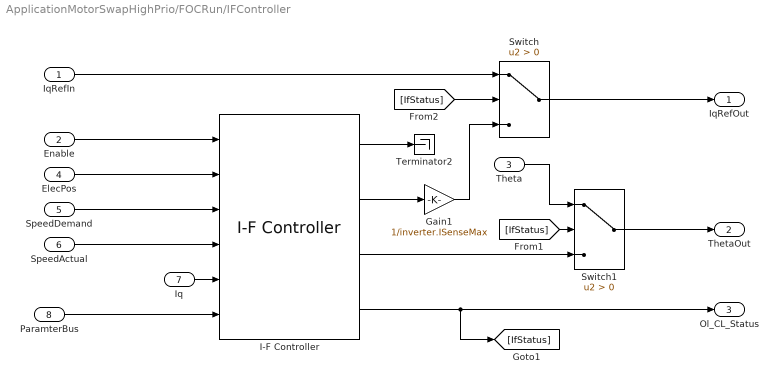
== system ApplicationMotorSwapHighPrio/FOCRun/IFController ==
  IqRefIn : Inport
  Enable : Inport  Port=2
  Theta : Inport  Port=3
  ElecPos : Inport  Port=4
  SpeedDemand : Inport  Port=5
  SpeedActual : Inport  Port=6
  Iq : Inport  Port=7
  ParamterBus : Inport  Port=8
  Gain1 : Gain  Gain=1/inverter.ISenseMax  RndMeth=Simplest  OutDataTypeStr=Inherit: Same as input
  I-F Controller : mcbpmsmiflib/I-F Controller  EnableSpeedDamp=off  PolePairs=4  PositionUnit=Per-unit  SpeedUnit=RPM  PerUnitSpeed=6000  CurrentUnit=SI unit  TempCurrentUnit=SI unit  MaxStatorCurrent=21.4286  BlkSampleTime=Ts  ParameterBusInput=on  OlClSpeed=400  ClOlSpeed=200  MaxStartingCurrent=7  MaxAcceleration=960  CurrentDownSlope=11  IdleTime=1  Angle=10 * pi / 180  VoltageUnit=SI unit  TempVoltageUnit=SI unit  MaxStatorVoltage=13.8564  DampCoeff=2.6172
  Switch : Switch  Criteria=u2 > Threshold  SaturateOnIntegerOverflow=off  InputSameDT=off
  Switch1 : Switch  Criteria=u2 > Threshold  SaturateOnIntegerOverflow=off  InputSameDT=off
  Terminator2 : Terminator
  IqRefOut : Outport
  ThetaOut : Outport  Port=2
  Ol_CL_Status : Outport  Port=3
  wires:
  IqRefIn/1 -> Switch/1
  ParamterBus/1 -> I-F Controller/6
  Switch/1 -> IqRefOut/1
  SpeedDemand/1 -> I-F Controller/3
  Switch1/1 -> ThetaOut/1
  SpeedActual/1 -> I-F Controller/4
  Iq/1 -> I-F Controller/5
  [IfStatus] -> Switch1/2
  I-F Controller/3 -> Switch1/3
  ElecPos/1 -> I-F Controller/2
  I-F Controller/4 -> [IfStatus], Ol_CL_Status/1
  I-F Controller/2 -> Gain1/1
  I-F Controller/1 -> Terminator2/1
  Theta/1 -> Switch1/1
  Enable/1 -> I-F Controller/1
  [IfStatus] -> Switch/2
  Gain1/1 -> Switch/3

== system ApplicationMotorSwapHighPrio/FluxObserver/Speed Calculation from Back EMF ==
  Vabc : Inport
  BusElementIn2 : Inport  Port=2  PortName=Config  Element=NRated
  BusElementIn3 : Inport  Port=2  PortName=Config  Element=P
  En : Inport  Port=3
  Demux : Demux  Outputs=3
  Speed Measurement : Subsystem
  Terminator : Terminator
  Vab_Speed : Outport
  wires:
  En/1 -> Speed Measurement/Enable
  Vabc/1 -> Demux/1
  Demux/2 -> Speed Measurement/2(Vb)
  Demux/1 -> Speed Measurement/1(Va)
  Speed Measurement/1(Speed) -> Vab_Speed/1
  BusElementIn3/1 -> Speed Measurement/4(p)
  Demux/3 -> Terminator/1
  BusElementIn2/1 -> Speed Measurement/3(SpeedRated)

== system ApplicationMotorSwapHighPrio/FluxObserver/Variant Subsystem ==
  Speed_FO : Inport
  Speed_Vabc : Inport  Port=2
  Ke : Inport  Port=3
  En : Inport  Port=4
  Codegen : Subsystem  VariantControl=(codegen)
  Sim : Subsystem  VariantControl=(sim)
  Speed : Outport

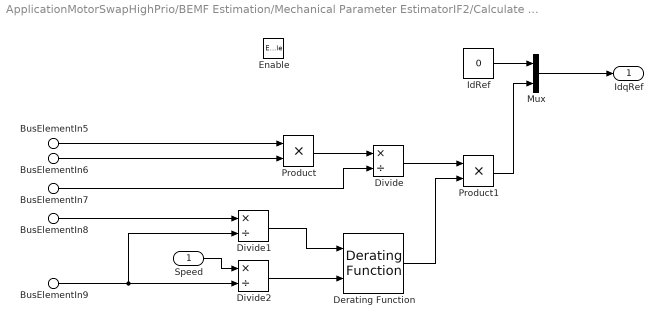
== system ApplicationMotorSwapHighPrio/BEMF Estimation/Mechanical Parameter EstimatorIF2/Calculate IqRef ==
  Speed : Inport
  BusElementIn5 : Inport  Port=2  PortName=Config  Element=IqRefFoc
  BusElementIn6 : Inport  Port=2  PortName=Config  Element=IRated
  BusElementIn7 : Inport  Port=2  PortName=Config  Element=ImaxInverter
  BusElementIn8 : Inport  Port=2  PortName=Config  Element=KeSpeed
  BusElementIn9 : Inport  Port=2  PortName=Config  Element=NRated
  Enable : EnablePort  StatesWhenEnabling=reset
  Derating Function : mcbcontrolslib/Derating Function  x=0.9
  Divide : Product  Inputs=*/  RndMeth=Simplest  OutDataTypeStr=Inherit: Same as first input
  Divide1 : Product  Inputs=*/  RndMeth=Simplest  OutDataTypeStr=Inherit: Same as first input
  Divide2 : Product  Inputs=*/  RndMeth=Simplest  OutDataTypeStr=Inherit: Same as first input
  IdRef : Constant  Value=0  OutDataTypeStr=single
  Mux : Mux  Inputs=2
  Product : Product  RndMeth=Simplest  OutDataTypeStr=Inherit: Same as first input
  Product1 : Product  RndMeth=Simplest  OutDataTypeStr=Inherit: Same as first input
  IdqRef : Outport
  wires:
  BusElementIn5/1 -> Product/1
  IdRef/1 -> Mux/1
  Mux/1 -> IdqRef/1
  BusElementIn6/1 -> Product/2
  Product/1 -> Divide/1
  BusElementIn7/1 -> Divide/2
  Divide/1 -> Product1/1
  Derating Function/1 -> Product1/2
  Speed/1 -> Divide2/1
  BusElementIn8/1 -> Divide1/1
  Divide1/1 -> Derating Function/1
  Divide2/1 -> Derating Function/2
  BusElementIn9/1 -> Divide1/2, Divide2/2
  Product1/1 -> Mux/2

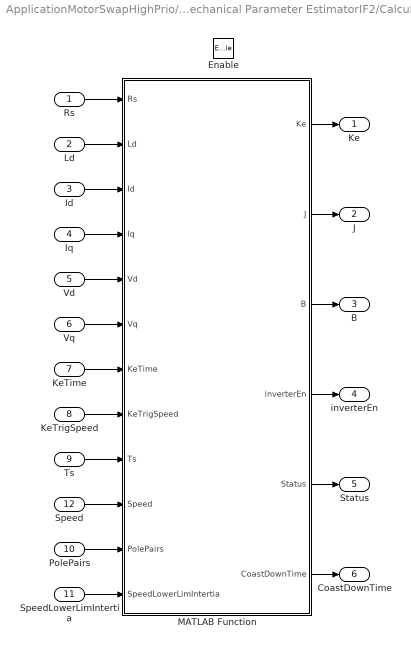
== system ApplicationMotorSwapHighPrio/BEMF Estimation/Mechanical Parameter EstimatorIF2/Calculate Parameters ==
  Rs : Inport
  Ld : Inport  Port=2
  Id : Inport  Port=3
  Iq : Inport  Port=4
  Vd : Inport  Port=5
  Vq : Inport  Port=6
  KeTime : Inport  Port=7
  KeTrigSpeed : Inport  Port=8
  Ts : Inport  Port=9
  PolePairs : Inport  Port=10
  SpeedLowerLimIntertia : Inport  Port=11
  Speed : Inport  Port=12
  Enable : EnablePort  StatesWhenEnabling=reset
  MATLAB Function : MATLAB Function  TreatAsAtomicUnit=on
  Ke : Outport
  J : Outport  Port=2
  B : Outport  Port=3
  inverterEn : Outport  Port=4  InitialOutput=1
  Status : Outport  Port=5  InitialOutput=1
  CoastDownTime : Outport  Port=6  InitialOutput=1
  wires:
  KeTrigSpeed/1 -> MATLAB Function/8(KeTrigSpeed)
  Speed/1 -> MATLAB Function/10(Speed)
  Ts/1 -> MATLAB Function/9(Ts)
  KeTime/1 -> MATLAB Function/7(KeTime)
  Vq/1 -> MATLAB Function/6(Vq)
  Vd/1 -> MATLAB Function/5(Vd)
  Iq/1 -> MATLAB Function/4(Iq)
  Id/1 -> MATLAB Function/3(Id)
  SpeedLowerLimIntertia/1 -> MATLAB Function/12(SpeedLowerLimIntertia)
  Ld/1 -> MATLAB Function/2(Ld)
  PolePairs/1 -> MATLAB Function/11(PolePairs)
  Rs/1 -> MATLAB Function/1(Rs)
  MATLAB Function/3(B) -> B/1
  MATLAB Function/1(Ke) -> Ke/1
  MATLAB Function/2(J) -> J/1
  MATLAB Function/4(inverterEn) -> inverterEn/1
  MATLAB Function/5(Status) -> Status/1
  MATLAB Function/6(CoastDownTime) -> CoastDownTime/1

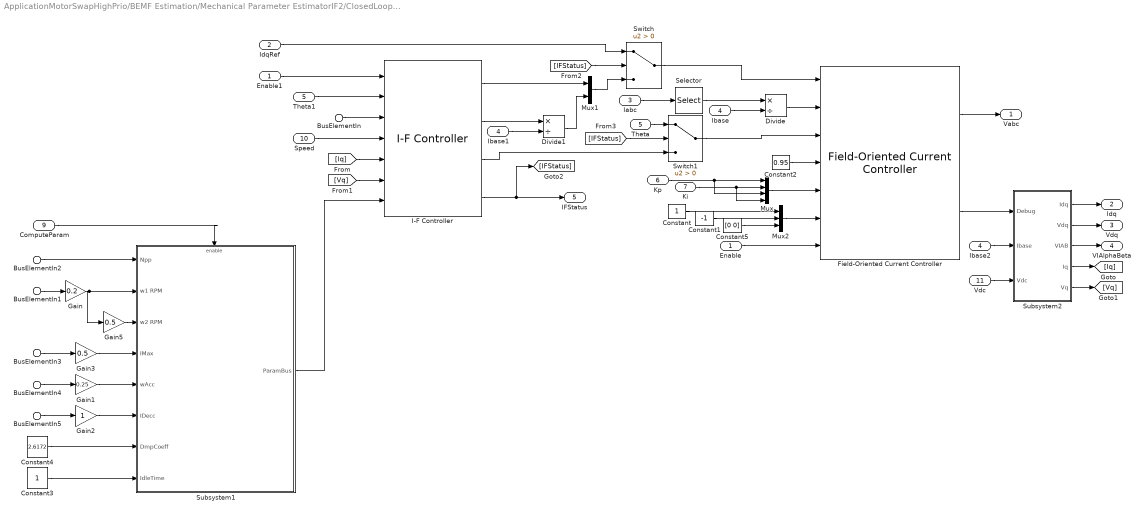
== system ApplicationMotorSwapHighPrio/BEMF Estimation/Mechanical Parameter EstimatorIF2/ClosedLoopFOC ==
  Enable : Inport
  IdqRef : Inport  Port=2
  Iabc : Inport  Port=3
  Ibase : Inport  Port=4
  Theta : Inport  Port=5
  Kp : Inport  Port=6
  Ki : Inport  Port=7
  BusElementIn : Inport  Port=8  PortName=Config  Element=KeSpeed
  BusElementIn1 : Inport  Port=8  PortName=Config  Element=NRated
  BusElementIn4 : Inport  Port=8  PortName=Config  Element=NRated
  BusElementIn2 : Inport  Port=8  PortName=Config  Element=P
  BusElementIn3 : Inport  Port=8  PortName=Config  Element=IRated
  BusElementIn5 : Inport  Port=8  PortName=Config  Element=IRated
  ComputeParam : Inport  Port=9
  Speed : Inport  Port=10
  Vdc : Inport  Port=11
  Constant : Constant  OutDataTypeStr=single
  Constant1 : Constant  Value=-1  OutDataTypeStr=single
  Constant2 : Constant  Value=0.95  OutDataTypeStr=single
  Constant3 : Constant  OutDataTypeStr=single
  Constant4 : Constant  Value=2.6172  OutDataTypeStr=single
  Constant5 : Constant  Value=[0 0]  OutDataTypeStr=single
  Divide : Product  Inputs=*/
  Divide1 : Product  Inputs=*/
  Enable1 : InportShadow
  Field-Oriented Current Controller : mcbfoclib/Field-Oriented Current Controller  AngleUnit=Per-unit  NumberOfLUTPoints=1024  AxisAlignment=D-axis  SaturationMethod=D-Q equivalence  PWMMethod=SVM: space vector modulation
  Gain : Gain  Gain=0.2  RndMeth=Simplest  OutDataTypeStr=Inherit: Same as input
  Gain1 : Gain  Gain=0.25  RndMeth=Simplest  OutDataTypeStr=Inherit: Same as input
  Gain2 : Gain  RndMeth=Simplest  OutDataTypeStr=Inherit: Same as input
  Gain3 : Gain  Gain=0.5  RndMeth=Simplest  OutDataTypeStr=Inherit: Same as input
  Gain5 : Gain  Gain=0.5  RndMeth=Simplest  OutDataTypeStr=Inherit: Same as input
  I-F Controller : mcbpmsmiflib/I-F Controller  EnableSpeedDamp=on  PolePairs=4  PositionUnit=Per-unit  SpeedUnit=RPM  PerUnitSpeed=6000  CurrentUnit=SI unit  TempCurrentUnit=SI unit  MaxStatorCurrent=21.4286  BlkSampleTime=Ts  ParameterBusInput=on  OlClSpeed=410.7  ClOlSpeed=287.49  MaxStartingCurrent=6.39  MaxAcceleration=960  CurrentDownSlope=111.8250  IdleTime=1  Angle=5 * 2 * pi / 360  VoltageUnit=SI unit  TempVoltageUnit=SI unit  MaxStatorVoltage=13.8564  DampCoeff=2.6172
  Ibase1 : InportShadow  Port=4
  Ibase2 : InportShadow  Port=4
  Mux : Mux
  Mux1 : Mux  Inputs=2
  Mux2 : Mux  Inputs=3
  Selector : Selector  InputPortWidth=3  IndexOptions=Index vector (dialog)  Indices=[1 2]  OutputSizes=1
  Subsystem1 : Subsystem
  Subsystem2 : Subsystem
  Switch : Switch  Criteria=u2 > Threshold  SaturateOnIntegerOverflow=off  InputSameDT=off
  Switch1 : Switch  Criteria=u2 > Threshold  SaturateOnIntegerOverflow=off  InputSameDT=off
  Theta1 : InportShadow  Port=5
  Vabc : Outport
  Idq : Outport  Port=2
  Vdq : Outport  Port=3
  VIAlphaBeta : Outport  Port=4
  IFStatus : Outport  Port=5
  wires:
  Mux/1 -> Field-Oriented Current Controller/5
  Ki/1 -> Mux/2, Mux/4
  Enable/1 -> Field-Oriented Current Controller/7
  Constant2/1 -> Field-Oriented Current Controller/4
  Constant1/1 -> Mux2/2
  Kp/1 -> Mux/1, Mux/3
  Field-Oriented Current Controller/1 -> Vabc/1
  Ibase/1 -> Divide/2
  Iabc/1 -> Selector/1
  Divide/1 -> Field-Oriented Current Controller/2
  Selector/1 -> Divide/1
  Constant/1 -> Mux2/1
  Constant5/1 -> Mux2/3
  Mux2/1 -> Field-Oriented Current Controller/6
  I-F Controller/1 -> Mux1/1
  Theta1/1 -> I-F Controller/2
  Enable1/1 -> I-F Controller/1
  BusElementIn/1 -> I-F Controller/3
  Mux1/1 -> Switch/3
  IdqRef/1 -> Switch/1
  Switch/1 -> Field-Oriented Current Controller/1
  I-F Controller/3 -> Switch1/3
  I-F Controller/4 -> [IFStatus], IFStatus/1
  Theta/1 -> Switch1/1
  Switch1/1 -> Field-Oriented Current Controller/3
  BusElementIn1/1 -> Gain/1
  BusElementIn4/1 -> Gain1/1
  BusElementIn5/1 -> Gain2/1
  BusElementIn2/1 -> Subsystem1/1(Npp)
  Gain/1 -> Gain5/1, Subsystem1/2(w1 RPM)
  BusElementIn3/1 -> Gain3/1
  Gain1/1 -> Subsystem1/5(wAcc)
  Gain2/1 -> Subsystem1/6(IDecc)
  Subsystem1/1(ParamBus) -> I-F Controller/7
  ComputeParam/1 -> Subsystem1/Enable
  Speed/1 -> I-F Controller/4
  Ibase1/1 -> Divide1/2
  I-F Controller/2 -> Divide1/1
  Divide1/1 -> Mux1/2
  Gain3/1 -> Subsystem1/4(IMax)
  Constant4/1 -> Subsystem1/7(DmpCoeff)
  Constant3/1 -> Subsystem1/8(IdleTime)
  Gain5/1 -> Subsystem1/3(w2 RPM)
  [Iq] -> I-F Controller/5
  [Vq] -> I-F Controller/6
  Field-Oriented Current Controller/2 -> Subsystem2/1(Debug)
  Ibase2/1 -> Subsystem2/2(Ibase)
  Vdc/1 -> Subsystem2/3(Vdc)
  Subsystem2/1(Idq) -> Idq/1
  Subsystem2/2(Vdq) -> Vdq/1
  Subsystem2/3(VIAB) -> VIAlphaBeta/1
  Subsystem2/4(Iq) -> [Iq]
  Subsystem2/5(Vq) -> [Vq]
  [IFStatus] -> Switch/2
  [IFStatus] -> Switch1/2

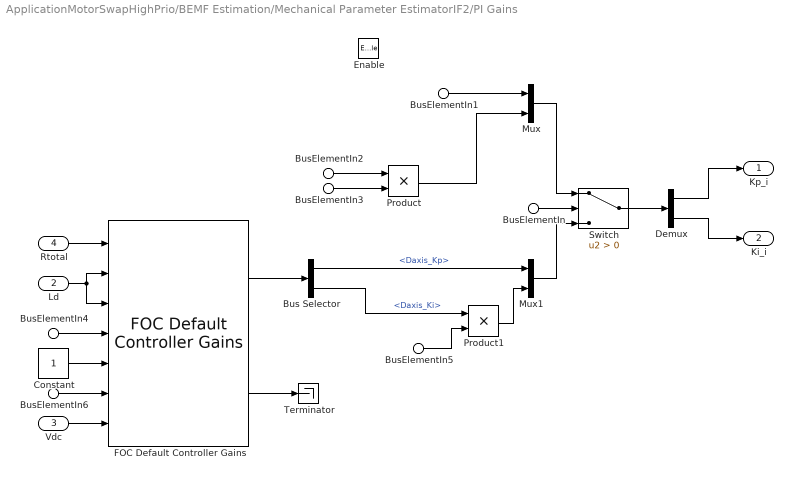
== system ApplicationMotorSwapHighPrio/BEMF Estimation/Mechanical Parameter EstimatorIF2/PI Gains ==
  BusElementIn1 : Inport  PortName=Config  Element=Kp
  BusElementIn2 : Inport  PortName=Config  Element=Ki
  BusElementIn3 : Inport  PortName=Config  Element=Ts
  BusElementIn5 : Inport  PortName=Config  Element=Ts
  BusElementIn4 : Inport  PortName=Config  Element=Ts
  BusElementIn : Inport  PortName=Config  Element=KpKiInputEnable
  BusElementIn6 : Inport  PortName=Config  Element=ImaxInverter
  Ld : Inport  Port=2  OutDataTypeStr=single
  Vdc : Inport  Port=3  OutDataTypeStr=single
  Rtotal : Inport  Port=4  OutDataTypeStr=single
  Enable : EnablePort
  Bus Selector : BusSelector  OutputSignals=Daxis_Kp,Daxis_Ki
  Constant : Constant  OutDataTypeStr=Inherit: Inherit via back propagation
  Demux : Demux  Outputs=2
  FOC Default Controller Gains : mcbcontrollergainlib/FOC Default Controller Gains  motorSelection=PMSM  unitType=Per-Unit  outCurrentControlGain=on  outFWCGain=off  outSpeedControlGain=off  externalDelay=off  currentSensorDelay=50e-6  speedSensorDelay=50e-6  speedFilterDelay=0.02
  Mux : Mux  Inputs=2
  Mux1 : Mux  Inputs=2
  Product : Product  RndMeth=Simplest  OutDataTypeStr=Inherit: Same as first input
  Product1 : Product  RndMeth=Simplest  OutDataTypeStr=Inherit: Same as first input
  Switch : Switch  Criteria=u2 > Threshold  SaturateOnIntegerOverflow=off  InputSameDT=off
  Terminator : Terminator
  Kp_i : Outport
  Ki_i : Outport  Port=2
  wires:
  FOC Default Controller Gains/2 -> Terminator/1
  BusElementIn/1 -> Switch/2
  Mux/1 -> Switch/1
  Switch/1 -> Demux/1
  Demux/1 -> Kp_i/1
  Demux/2 -> Ki_i/1
  BusElementIn1/1 -> Mux/1
  BusElementIn2/1 -> Product/1
  BusElementIn3/1 -> Product/2
  Product/1 -> Mux/2
  Mux1/1 -> Switch/3
  Bus Selector/1 -> Mux1/1  "<Daxis_Kp>"
  Bus Selector/2 -> Product1/1  "<Daxis_Ki>"
  Product1/1 -> Mux1/2
  BusElementIn5/1 -> Product1/2
  Rtotal/1 -> FOC Default Controller Gains/1
  Ld/1 -> FOC Default Controller Gains/3, FOC Default Controller Gains/2
  BusElementIn4/1 -> FOC Default Controller Gains/4
  Vdc/1 -> FOC Default Controller Gains/7
  BusElementIn6/1 -> FOC Default Controller Gains/6
  Constant/1 -> FOC Default Controller Gains/5
  FOC Default Controller Gains/1 -> Bus Selector/1

== system ApplicationMotorSwapHighPrio/BEMF Estimation/Mechanical Parameter EstimatorIF2/Test Control Stateflow ==
  StartEst : Inport
  StartFOC : Inport  Port=2
  InvEn : Inport  Port=3
  StatusIn : Inport  Port=4
  BusElementIn : Inport  Port=5  PortName=Config  Element=Ts
  BusElementIn1 : Inport  Port=5  PortName=Config  Element=KeTime
  Data Type Conversion : DataTypeConversion  OutDataTypeStr=boolean  RndMeth=Simplest  SaturateOnIntegerOverflow=off
  Data Type Conversion1 : DataTypeConversion  OutDataTypeStr=boolean  RndMeth=Simplest  SaturateOnIntegerOverflow=off
  Stateflow : Stateflow chart  TreatAsAtomicUnit=on
  Unit Delay : UnitDelay  SampleTime=-1  HasFrameUpgradeWarning=on
  VabcEn : Outport
  ClosedLoopEn : Outport  Port=2
  CalcParams : Outport  Port=3
  PIGainEn : Outport  Port=4
  StatusOut : Outport  Port=5
  wires:
  Stateflow/4(PIGainEn) -> PIGainEn/1
  StartEst/1 -> Data Type Conversion/1
  StartFOC/1 -> Data Type Conversion1/1
  Data Type Conversion/1 -> Unit Delay/1, Stateflow/1(EnIn)
  Unit Delay/1 -> Stateflow/2(EnInPrev)
  Data Type Conversion1/1 -> Stateflow/3(StartFOC)
  InvEn/1 -> Stateflow/4(InvEn)
  StatusIn/1 -> Stateflow/5(StatusIn)
  BusElementIn1/1 -> Stateflow/6(KeTime)
  BusElementIn/1 -> Stateflow/7(Ts)
  Stateflow/1(VabcEn) -> VabcEn/1
  Stateflow/2(ClosedLoopEn) -> ClosedLoopEn/1
  Stateflow/5(StatusOut) -> StatusOut/1
  Stateflow/3(CalcParams) -> CalcParams/1

== system ApplicationMotorSwapHighPrio/BEMF Estimation/Select J/Codegen ==
  J In : Inport
  J Out : Outport
  wires:
  J In/1 -> J Out/1

== system ApplicationMotorSwapHighPrio/BEMF Estimation/Select J/Sim ==
  J In : Inport
  Constant : Constant  Value=pmsm.J  OutDataTypeStr=dataType
  Terminator : Terminator
  J Out : Outport
  wires:
  Constant/1 -> J Out/1
  J In/1 -> Terminator/1

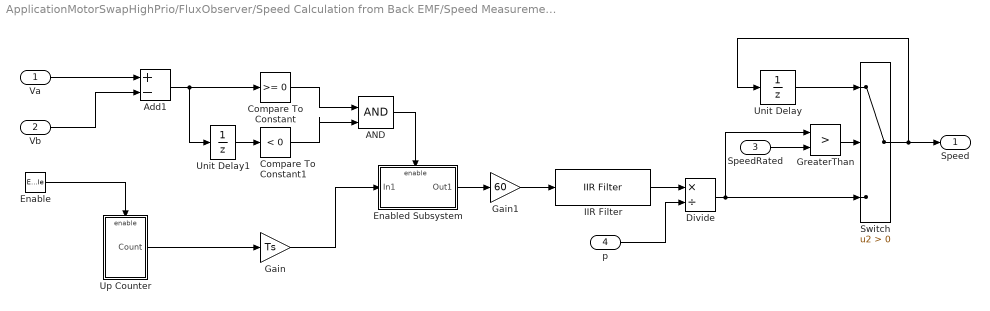
== system ApplicationMotorSwapHighPrio/FluxObserver/Speed Calculation from Back EMF/Speed Measurement ==
  Va : Inport
  Vb : Inport  Port=2
  SpeedRated : Inport  Port=3
  p : Inport  Port=4
  Enable : EnablePort  StatesWhenEnabling=reset  ShowOutputPort=on
  AND : Logic  IconShape=distinctive  AllPortsSameDT=off  OutDataTypeStr=boolean
  Add1 : Sum  Inputs=+-
  Compare To Constant : simulink/Logic and Bit Operations/Compare To Constant  relop=>=  const=0  OutDataTypeStr=boolean
  Compare To Constant1 : simulink/Logic and Bit Operations/Compare To Constant  relop=<  const=0  OutDataTypeStr=boolean
  Divide : Product  Inputs=*/
  Enabled Subsystem : Subsystem  TreatAsAtomicUnit=on
  Gain : Gain  Gain=Ts  OutDataTypeStr=dataType  RndMeth=Simplest
  Gain1 : Gain  Gain=60  RndMeth=Simplest  OutDataTypeStr=Inherit: Same as input
  GreaterThan : RelationalOperator  Operator=>  OutDataTypeStr=boolean  RndMeth=Simplest  InputSameDT=off
  IIR Filter : mcbcontrolslib/IIR Filter  VariantControl=Low Pass Filter  VariantSelect=Low-pass  FilterConstantInputType=Specify via dialog  Filter_constant=0.01  advancedSettings=on  Ts=Ts  cutOff_freq=25.722
  Switch : Switch  Criteria=u2 > Threshold  SaturateOnIntegerOverflow=off  InputSameDT=off
  Unit Delay : UnitDelay  SampleTime=-1  HasFrameUpgradeWarning=on
  Unit Delay1 : UnitDelay  SampleTime=-1  HasFrameUpgradeWarning=on
  Up Counter : Subsystem
  Speed : Outport  OutputWhenDisabled=reset  InitialOutput=0
  wires:
  IIR Filter/1 -> Divide/1
  Vb/1 -> Add1/2
  Compare To Constant/1 -> AND/1
  Add1/1 -> Compare To Constant/1, Unit Delay1/1
  Compare To Constant1/1 -> AND/2
  Unit Delay1/1 -> Compare To Constant1/1
  Enabled Subsystem/1(Out1) -> Gain1/1
  Gain1/1 -> IIR Filter/1
  AND/1 -> Enabled Subsystem/Enable
  Gain/1 -> Enabled Subsystem/1(In1)
  Va/1 -> Add1/1
  Up Counter/1(Count) -> Gain/1
  Enable/1 -> Up Counter/Enable
  Switch/1 -> Unit Delay/1, Speed/1
  Divide/1 -> GreaterThan/1, Switch/3
  Unit Delay/1 -> Switch/1
  GreaterThan/1 -> Switch/2
  SpeedRated/1 -> GreaterThan/2
  p/1 -> Divide/2

== system ApplicationMotorSwapHighPrio/FluxObserver/Variant Subsystem/Codegen ==
  Speed_Vabc : Inport
  Speed_FO : Inport  Port=2
  Ke : Inport  Port=3
  En : Inport  Port=4
  AND : Logic  IconShape=distinctive  AllPortsSameDT=off  OutDataTypeStr=boolean
  Compare To Constant2 : simulink/Logic and Bit Operations/Compare To Constant  relop=>  const=0  OutDataTypeStr=boolean
  Switch : Switch  Criteria=u2 > Threshold  SaturateOnIntegerOverflow=off  InputSameDT=off
  Speed : Outport
  wires:
  Switch/1 -> Speed/1
  AND/1 -> Switch/2
  Compare To Constant2/1 -> AND/1
  Ke/1 -> Compare To Constant2/1
  Speed_Vabc/1 -> Switch/1
  Speed_FO/1 -> Switch/3
  En/1 -> AND/2

== system ApplicationMotorSwapHighPrio/FluxObserver/Variant Subsystem/Sim ==
  Speed_Vabc : Inport
  Speed_FO : Inport  Port=2
  Ke : Inport  Port=3
  En : Inport  Port=4
  Terminator : Terminator
  Terminator1 : Terminator
  Terminator2 : Terminator
  Speed : Outport
  wires:
  Ke/1 -> Terminator1/1
  Speed_Vabc/1 -> Terminator/1
  Speed_FO/1 -> Speed/1
  En/1 -> Terminator2/1
